simulink model "Ex_5"  (Simulink 8.0)
settings: Solver=ode45  StartTime=0.0  StopTime=10.0  RelTol=1e-3
settings Model: Creator=Faradars  LastModifiedBy=Faradars

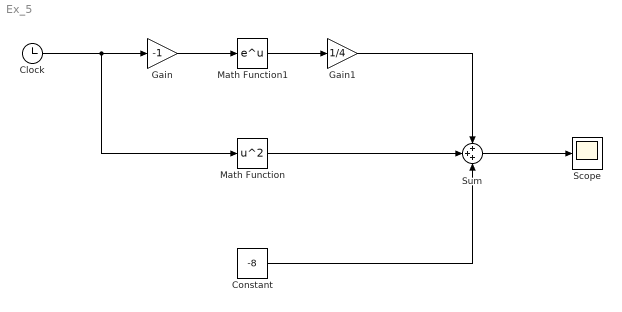
== system Ex_5 ==
  Clock : Clock
  Constant : Constant  Value=-8
  Gain : Gain  Gain=-1
  Gain1 : Gain  Gain=1/4
  Math Function : Math  Operator=square  SaturateOnIntegerOverflow=on
  Math Function1 : Math  SaturateOnIntegerOverflow=on
  Scope : Scope
  Sum : Sum  Inputs=+++
  wires:
  Clock/1 -> Math Function/1, Gain/1
  Gain/1 -> Math Function1/1
  Math Function1/1 -> Gain1/1
  Math Function/1 -> Sum/2
  Gain1/1 -> Sum/1
  Constant/1 -> Sum/3
  Sum/1 -> Scope/1
